simulink subsystem "Full_Bore_Ball_Valve"  (R2020b)
settings: Solver=VariableStepAuto  StartTime=0.0  StopTime=10.0  RelTol=1e-3
model mask{Cv=0.5, portCrossSection=2e-5}
  mask prompts: Cv "Cv Flow Coefficient when fully open (Imperial Units)"; portCrossSection "Cross-sectional area at ports A and B (m^2):"
libraries: nesl_utility x2, SimscapeCustomBlocks_lib x1
settings Model: Creator=Edward  LastModifiedBy=Edward

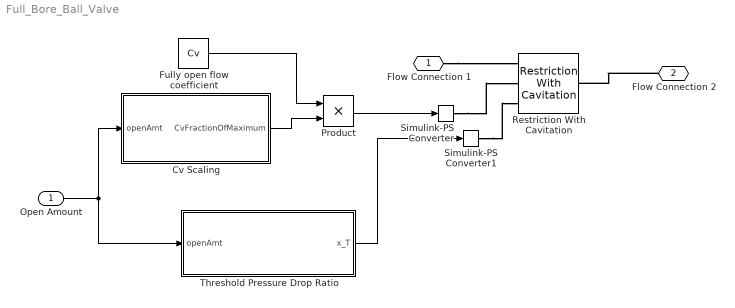
== system Full_Bore_Ball_Valve ==
  Open Amount : Inport
  Cv Scaling : MATLAB Function  TreatAsAtomicUnit=on
  Fully open flow coefficient : Constant  Value=Cv
  Product : Product
  Restriction With Cavitation : SimscapeCustomBlocks_lib/Restriction With Cavitation  area=portCrossSection m^2  F_L=0.45  F_d=1  X_liquid_threshold=0.6  X_gas_theshold=0.9
      settings: InternalSimscapePortConfiguration="{\"Bottom\":[],\"Left\":[{\"id\":\"A\",\"label\":\"A\",\"type\":\"foundation.two_phase_fluid.two_phase_fluid\"},{\"id\":\"Cv\",\"label\":\"Cv\",\"type\":\"input\"},{\"id\":\"x_T\",\"label\":\"x_T\",\"type\":\"input\"}],\"Right\":[{\"id\":\"B\",\"label\":\"B\",\"type\":\"foundation.two_phase_fluid.two_phase_fluid\"}],\"Top\":[]}"
  Simulink-PS Converter : nesl_utility/Simulink-PS Converter  PhysicalDomain=network_engine_domain  SubClassName=ps_input  LeftPortType=input  RightPortType=output  PseudoPeriodic=off  Frequencies=[]  NoiseDistribution=none  NoiseParameters=[]  Unit=1  AffineConversion=off  FilteringAndDerivatives=provide  SimscapeFilterOrder=1  InputFilterTimeConstant=0.001  UdotUserProvided=0
  Simulink-PS Converter1 : nesl_utility/Simulink-PS Converter  PhysicalDomain=network_engine_domain  SubClassName=ps_input  LeftPortType=input  RightPortType=output  PseudoPeriodic=off  Frequencies=[]  NoiseDistribution=none  NoiseParameters=[]  Unit=1  AffineConversion=off  FilteringAndDerivatives=provide  SimscapeFilterOrder=1  InputFilterTimeConstant=0.001  UdotUserProvided=0
  Threshold Pressure Drop Ratio : MATLAB Function  TreatAsAtomicUnit=on
  Flow Connection 1 : PMIOPort  Side=Left
  Flow Connection 2 : PMIOPort  Port=2  Side=Right
  wires:
  Threshold Pressure Drop Ratio/1(x_T) -> Simulink-PS Converter1/1
  Open Amount/1 -> Threshold Pressure Drop Ratio/1(openAmt), Cv Scaling/1(openAmt)
  Product/1 -> Simulink-PS Converter/1
  Cv Scaling/1(CvFractionOfMaximum) -> Product/2
  Fully open flow coefficient/1 -> Product/1
  connections:
  Flow Connection 1/RConn1 -- Restriction With Cavitation/LConn1
  Simulink-PS Converter/RConn1 -- Restriction With Cavitation/LConn2
  Simulink-PS Converter1/RConn1 -- Restriction With Cavitation/LConn3
  Flow Connection 2/RConn1 -- Restriction With Cavitation/RConn1

== matlab function Full_Bore_Ball_Valve/Threshold Pressure Drop Ratio ==
  data: openAmt input; x_T output
function x_T = thresholdPressureDropRatioFactor(openAmt)
%Col1: open amount (0->1), Col2: Threshold pressure drop ratio factor x_T
assert(openAmt>=0 && openAmt<=1, 'Opening amount must be between 0 and 1');
%Raw data taken for ball valve type from graph from
%https://www.valin.com/resources/blog/gas-flow-control-valves
rawData = [0, 0.6389830508474577
0.09604519774011297, 0.6389830508474577
0.19689265536723163, 0.6406779661016949
0.2759887005649718, 0.6338983050847458
0.457909604519774, 0.6000000000000001
0.6951977401129945, 0.4915254237288136
0.8909604519774011, 0.32372881355932204
1, 0.15932203389830513];
x_T = interp1(rawData(:,1), rawData(:,2), openAmt, 'spline');

== matlab function Full_Bore_Ball_Valve/Cv Scaling ==
  data: openAmt input; CvFractionOfMaximum output
function CvFractionOfMaximum = CvScaling(openAmt)
%Polynomial fit for typical full bore ball valve Cv as fraction of maximum
%for open amount between 0 and 1
P = [-8.20125000000194	15.4351730769290	-8.93336538462210	2.68560314685672	-0.247832167833044	0.259200466200549	0];
assert(openAmt>=0 && openAmt<=1, 'Opening amount must be between 0 and 1');
CvFractionOfMaximum = polyval(P, openAmt);
